simulink model "model_samochodu"  (Simulink 8.5)
settings: Solver=ode45  SolverMode=SingleTasking  StartTime=0.0  StopTime=40.0  RelTol=1e-3
values from neighbouring files (symbols this model uses):
  Af = 1.63    [Car_Model.m]
  alpha = 1000    [Car_Model.m]
  c_ad = 0.418    [Car_Model.m]
  g = 9.81    [Car_Model.m]
  J_eng = 0.5    [Car_Model.m]
  J_wh = 0.75    [Car_Model.m]
  Lrr = 0.282    [Car_Model.m]
  m_v = 800    [Car_Model.m]
  r_fdr = 4.07    [Car_Model.m]
  r_g = 2.038    [Car_Model.m]
  ro = 1.2    [Car_Model.m]
  tau_brk = 0.05    [Car_Model.m]
  tau_pwr = 0.2    [Car_Model.m]
  Tbrk = 0    [Car_Model.m]
  Tpwr = 1450    [Car_Model.m]
  v_zero = 0    [Car_Model.m]
settings Model: Creator=eve-1  LastModifiedBy=Michas  CovMetricSettings=dwe  CovHtmlReporting=off  covSaveCumulativeToWorkspaceVar=off  CovSaveSingleToWorkspaceVar=off  CovExternalEMLEnable=on
settings DataIOCC: LimitDataPoints=off  SaveFormat=Dataset  SignalLoggingSaveFormat=Dataset
settings OptimizationCC: ExpressionDepthLimit=128
settings DebuggingCC: UnderspecifiedInitializationDetection=Simplified  MergeDetectMultiDrivingBlocksExec=error  FcnCallInpInsideContextMsg=EnableAllAsError  StateNameClashWarn=none  SFUnexpectedBacktrackingDiag=error  SFNoUnconditionalDefaultTransitionDiag=error
settings HardwareCC: ProdBitPerPointer=64  ProdLargestAtomicFloat=Float  ProdIntDivRoundTo=Zero  ProdEndianess=LittleEndian  ProdHWDeviceType=Specified
settings ModelReferenceCC: PropagateSignalLabelsOutOfModel=on
settings GRTTargetCC: TargetLangStandard=C99 (ISO)  GeneratePreprocessorConditionals=Use local settings  CombineOutputUpdateFcns=on  GRTInterface=off

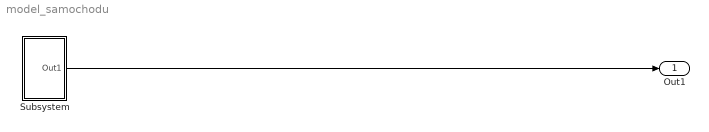
== system model_samochodu ==
  Subsystem : Subsystem
  Out1 : Outport
  wires:
  Subsystem/1(Out1) -> Out1/1

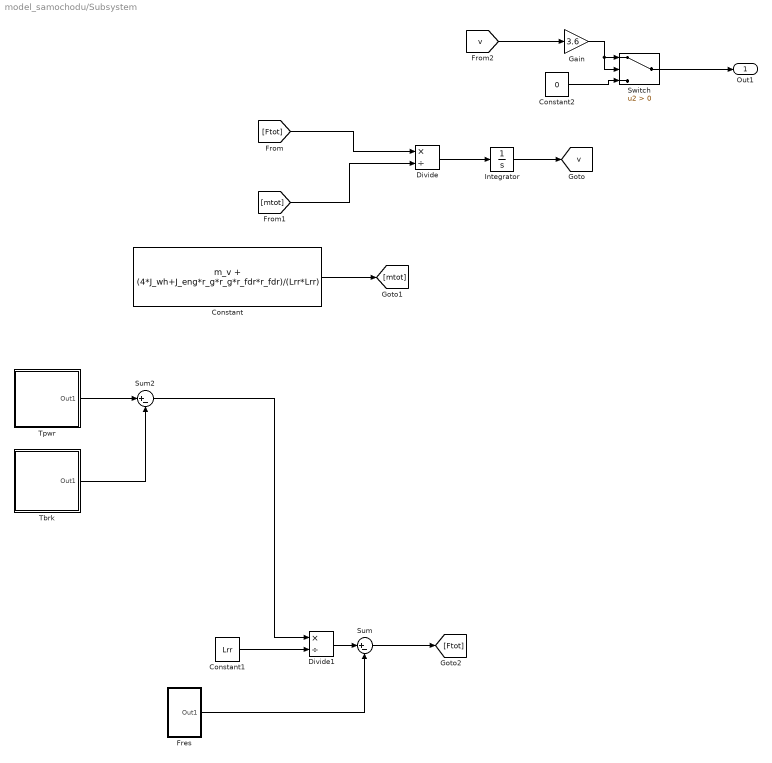
== system model_samochodu/Subsystem ==
  Constant : Constant  Value=m_v + (4*J_wh+J_eng*r_g*r_g*r_fdr*r_fdr)/(Lrr*Lrr)
  Constant1 : Constant  Value=Lrr
  Constant2 : Constant  Value=0
  Divide : Product  Inputs=*/
  Divide1 : Product  Inputs=*/
  Fres : Subsystem
  Gain : Gain  Gain=3.6
  Integrator : Integrator  InitialCondition=v_zero
  Sum : Sum  Inputs=|+-
  Sum2 : Sum  Inputs=|+-
  Switch : Switch  Criteria=u2 > Threshold
  Tbrk : Subsystem
  Tpwr : Subsystem
  Out1 : Outport
  tag scope: v=global
  wires:
  Constant1/1 -> Divide1/2
  [v] -> Gain/1
  Divide1/1 -> Sum/1
  Sum/1 -> [Ftot]
  Fres/1(Out1) -> Sum/2
  Tpwr/1(Out1) -> Sum2/1
  [mtot] -> Divide/2
  Tbrk/1(Out1) -> Sum2/2
  Divide/1 -> Integrator/1
  Integrator/1 -> [v]
  Sum2/1 -> Divide1/1
  [Ftot] -> Divide/1
  Constant/1 -> [mtot]
  Constant2/1 -> Switch/3
  Gain/1 -> Switch/1, Switch/2
  Switch/1 -> Out1/1

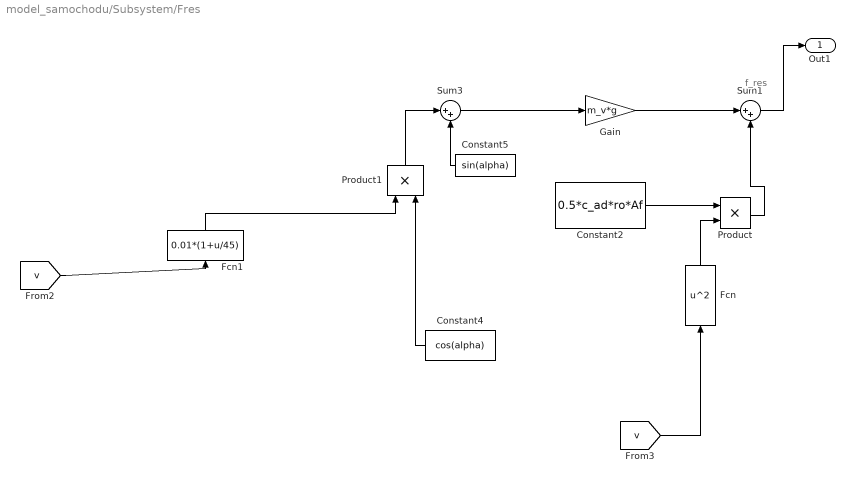
== system model_samochodu/Subsystem/Fres ==
  note: f_res
  Constant2 : Constant  Value=0.5*c_ad*ro*Af
  Constant4 : Constant  Value=cos(alpha)
  Constant5 : Constant  Value=sin(alpha)
  Fcn : Fcn  Expr=u^2
  Fcn1 : Fcn  Expr=0.01*(1+u/45)
  Gain : Gain  Gain=m_v*g
  Product : Product
  Product1 : Product
  Sum1 : Sum  Inputs=|++
  Sum3 : Sum  Inputs=|++
  Out1 : Outport
  wires:
  [v] -> Fcn1/1
  [v] -> Fcn/1
  Constant5/1 -> Sum3/2
  Gain/1 -> Sum1/1
  Product/1 -> Sum1/2
  Constant4/1 -> Product1/2
  Sum3/1 -> Gain/1
  Sum1/1 -> Out1/1
  Product1/1 -> Sum3/1
  Fcn1/1 -> Product1/1
  Fcn/1 -> Product/2
  Constant2/1 -> Product/1

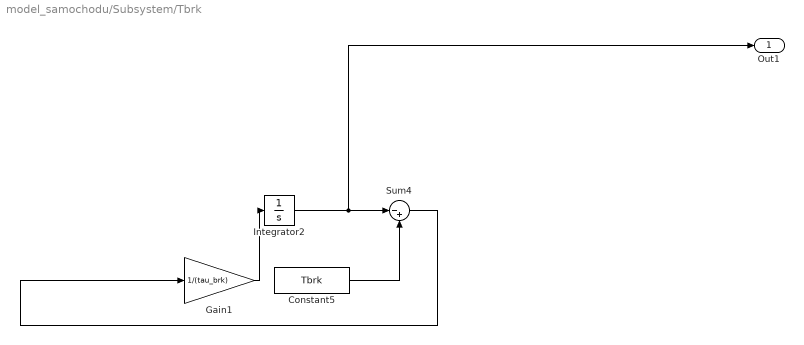
== system model_samochodu/Subsystem/Tbrk ==
  Constant5 : Constant  Value=Tbrk
  Gain1 : Gain  Gain=1/(tau_brk)
  Integrator2 : Integrator
  Sum4 : Sum  Inputs=|-+
  Out1 : Outport
  wires:
  Sum4/1 -> Gain1/1
  Integrator2/1 -> Out1/1, Sum4/1
  Constant5/1 -> Sum4/2
  Gain1/1 -> Integrator2/1

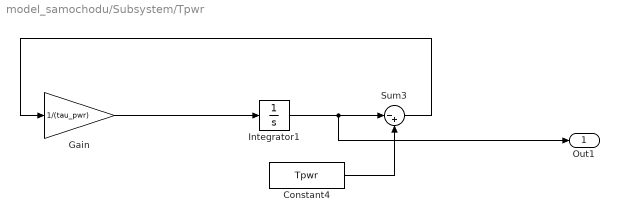
== system model_samochodu/Subsystem/Tpwr ==
  Constant4 : Constant  Value=Tpwr
  Gain : Gain  Gain=1/(tau_pwr)
  Integrator1 : Integrator
  Sum3 : Sum  Inputs=|-+
  Out1 : Outport
  wires:
  Gain/1 -> Integrator1/1
  Integrator1/1 -> Out1/1, Sum3/1
  Constant4/1 -> Sum3/2
  Sum3/1 -> Gain/1
